simulink model "VCU_CS75_12_27_test"  (R2014a)
settings: Solver=FixedStepDiscrete  StartTime=0.0  StopTime=25  FixedStep=0.0005  RelTol=1e-3
undefined symbols (not defined in the file): D1, D2, D3, ecucoder_acal, ErrorSumMax1, ErrorSumMax2, ErrorSumMax3, I1, I2, I3, I_SW01_L, LaterlAngleCommand, LDW, P1, P2, P3, RemoteAcclPosition
libraries: simulink x913, ec5744lib x39
(part 27 of 30)

== system VCU_CS75_12_27_test/长安CS75底盘程序，20ms一次/Input/CAN1_Rx/ESP_281/ReceiveMessages/Subsystem/ESP_2 ==
  input : Inport
  Demux : Demux  Outputs=8
  ESP_ABSActiveStatus_Ad : Sum
  ESP_ABSActiveStatus_Convert : DataTypeConversion  OutDataTypeStr=uint32
  ESP_ABSActiveStatus_F : Gain
  ESP_ABSActiveStatus_L : simulink/Logic and Bit Operations/Bitwise Operator  logicop=AND  UseBitMask=on  BitMask=128  BitMaskRealWorld=Stored Integer
  ESP_ABSActiveStatus_O : Constant  Value=0  OutDataTypeStr=single
  ESP_ABSActiveStatus_S : ArithShift  BitShiftNumber=7
  ESP_ABSActiveStatus_Sub : Subsystem
  ESP_ABSActiveStatus_sat : Saturate  UpperLimit=1  LowerLimit=0
  ESP_ABSActiveStatuscv : DataTypeConversion
  ESP_ABSFailStatus_Ad : Sum
  ESP_ABSFailStatus_Convert : DataTypeConversion  OutDataTypeStr=uint32
  ESP_ABSFailStatus_F : Gain
  ESP_ABSFailStatus_L : simulink/Logic and Bit Operations/Bitwise Operator  logicop=AND  UseBitMask=on  BitMask=8  BitMaskRealWorld=Stored Integer
  ESP_ABSFailStatus_O : Constant  Value=0  OutDataTypeStr=single
  ESP_ABSFailStatus_S : ArithShift  BitShiftNumber=3
  ESP_ABSFailStatus_Sub : Subsystem
  ESP_ABSFailStatus_sat : Saturate  UpperLimit=1  LowerLimit=0
  ESP_ABSFailStatuscv : DataTypeConversion
  ESP_BrakePedalStatus_Ad : Sum
  ESP_BrakePedalStatus_Convert : DataTypeConversion  OutDataTypeStr=uint32
  ESP_BrakePedalStatus_F : Gain
  ESP_BrakePedalStatus_L : simulink/Logic and Bit Operations/Bitwise Operator  logicop=AND  UseBitMask=on  BitMask=96  BitMaskRealWorld=Stored Integer
  ESP_BrakePedalStatus_O : Constant  Value=0  OutDataTypeStr=single
  ESP_BrakePedalStatus_S : ArithShift  BitShiftNumber=5
  ESP_BrakePedalStatus_Sub : Subsystem
  ESP_BrakePedalStatus_sat : Saturate  UpperLimit=3  LowerLimit=0
  ESP_BrakePedalStatuscv : DataTypeConversion
  ESP_Checksum_Ad : Sum
  ESP_Checksum_Convert : DataTypeConversion  OutDataTypeStr=uint32
  ESP_Checksum_F : Gain
  ESP_Checksum_L : simulink/Logic and Bit Operations/Bitwise Operator  logicop=AND  UseBitMask=on  BitMask=255  BitMaskRealWorld=Stored Integer
  ESP_Checksum_O : Constant  Value=0  OutDataTypeStr=single
  ESP_Checksum_S : ArithShift
  ESP_Checksum_Sub : Subsystem
  ESP_Checksum_sat : Saturate  UpperLimit=255  LowerLimit=0
  ESP_Checksumcv : DataTypeConversion
  ESP_EBDFailStatus_Ad : Sum
  ESP_EBDFailStatus_Convert : DataTypeConversion  OutDataTypeStr=uint32
  ESP_EBDFailStatus_F : Gain
  ESP_EBDFailStatus_L : simulink/Logic and Bit Operations/Bitwise Operator  logicop=AND  UseBitMask=on  BitMask=4  BitMaskRealWorld=Stored Integer
  ESP_EBDFailStatus_O : Constant  Value=0  OutDataTypeStr=single
  ESP_EBDFailStatus_S : ArithShift  BitShiftNumber=2
  ESP_EBDFailStatus_Sub : Subsystem
  ESP_EBDFailStatus_sat : Saturate  UpperLimit=1  LowerLimit=0
  ESP_EBDFailStatuscv : DataTypeConversion
  ESP_ESPActiveStatus_Ad : Sum
  ESP_ESPActiveStatus_Convert : DataTypeConversion  OutDataTypeStr=uint32
  ESP_ESPActiveStatus_F : Gain
  ESP_ESPActiveStatus_L : simulink/Logic and Bit Operations/Bitwise Operator  logicop=AND  UseBitMask=on  BitMask=1  BitMaskRealWorld=Stored Integer
  ESP_ESPActiveStatus_O : Constant  Value=0  OutDataTypeStr=single
  ESP_ESPActiveStatus_S : ArithShift
  ESP_ESPActiveStatus_Sub : Subsystem
  ESP_ESPActiveStatus_sat : Saturate  UpperLimit=1  LowerLimit=0
  ESP_ESPActiveStatuscv : DataTypeConversion
  ESP_ESPFailStatus_Ad : Sum
  ESP_ESPFailStatus_Convert : DataTypeConversion  OutDataTypeStr=uint32
  ESP_ESPFailStatus_F : Gain
  ESP_ESPFailStatus_L : simulink/Logic and Bit Operations/Bitwise Operator  logicop=AND  UseBitMask=on  BitMask=16  BitMaskRealWorld=Stored Integer
  ESP_ESPFailStatus_O : Constant  Value=0  OutDataTypeStr=single
  ESP_ESPFailStatus_S : ArithShift  BitShiftNumber=4
  ESP_ESPFailStatus_Sub : Subsystem
  ESP_ESPFailStatus_sat : Saturate  UpperLimit=1  LowerLimit=0
  ESP_ESPFailStatuscv : DataTypeConversion
  ESP_ESPSwitchStatus_Ad : Sum
  ESP_ESPSwitchStatus_Convert : DataTypeConversion  OutDataTypeStr=uint32
  ESP_ESPSwitchStatus_F : Gain
  ESP_ESPSwitchStatus_L : simulink/Logic and Bit Operations/Bitwise Operator  logicop=AND  UseBitMask=on  BitMask=2  BitMaskRealWorld=Stored Integer
  ESP_ESPSwitchStatus_O : Constant  Value=0  OutDataTypeStr=single
  ESP_ESPSwitchStatus_S : ArithShift  BitShiftNumber=1
  ESP_ESPSwitchStatus_Sub : Subsystem
  ESP_ESPSwitchStatus_sat : Saturate  UpperLimit=1  LowerLimit=0
  ESP_ESPSwitchStatuscv : DataTypeConversion
  ESP_RollingCounter_Ad : Sum
  ESP_RollingCounter_Convert : DataTypeConversion  OutDataTypeStr=uint32
  ESP_RollingCounter_F : Gain
  ESP_RollingCounter_L : simulink/Logic and Bit Operations/Bitwise Operator  logicop=AND  UseBitMask=on  BitMask=15  BitMaskRealWorld=Stored Integer
  ESP_RollingCounter_O : Constant  Value=0  OutDataTypeStr=single
  ESP_RollingCounter_S : ArithShift
  ESP_RollingCounter_Sub : Subsystem
  ESP_RollingCounter_sat : Saturate  UpperLimit=15  LowerLimit=0
  ESP_RollingCountercv : DataTypeConversion
  ESP_VehicleSpeed_Ad : Sum
  ESP_VehicleSpeed_Convert : DataTypeConversion  OutDataTypeStr=uint32
  ESP_VehicleSpeed_F : Gain  Gain=0.05625
  ESP_VehicleSpeed_L : simulink/Logic and Bit Operations/Bitwise Operator  logicop=AND  UseBitMask=on  BitMask=8191  BitMaskRealWorld=Stored Integer
  ESP_VehicleSpeed_O : Constant  Value=0  OutDataTypeStr=single
  ESP_VehicleSpeed_S : ArithShift
  ESP_VehicleSpeed_Status_Ad : Sum
  ESP_VehicleSpeed_Status_Convert : DataTypeConversion  OutDataTypeStr=uint32
  ESP_VehicleSpeed_Status_F : Gain
  ESP_VehicleSpeed_Status_L : simulink/Logic and Bit Operations/Bitwise Operator  logicop=AND  UseBitMask=on  BitMask=32  BitMaskRealWorld=Stored Integer
  ESP_VehicleSpeed_Status_O : Constant  Value=0  OutDataTypeStr=single
  ESP_VehicleSpeed_Status_S : ArithShift  BitShiftNumber=5
  ESP_VehicleSpeed_Status_Sub : Subsystem
  ESP_VehicleSpeed_Status_sat : Saturate  UpperLimit=1  LowerLimit=0
  ESP_VehicleSpeed_Statuscv : DataTypeConversion
  ESP_VehicleSpeed_Sub : Subsystem
  ESP_VehicleSpeed_sat : Saturate  UpperLimit=360  LowerLimit=0
  ESP_VehicleSpeedcv : DataTypeConversion
  ESP_VehicleSpeedinput5_Ad : Sum
  ESP_VehicleSpeedinput5_C : Constant  Value=256
  ESP_VehicleSpeedinput5_P : Product
  ESP_ESPActiveStatus_Out : Outport
  ESP_ESPSwitchStatus_Out : Outport  Port=2
  ESP_EBDFailStatus_Out : Outport  Port=3
  ESP_ABSFailStatus_Out : Outport  Port=4
  ESP_ESPFailStatus_Out : Outport  Port=5
  ESP_ABSActiveStatus_Out : Outport  Port=6
  ESP_VehicleSpeed_Out : Outport  Port=7
  ESP_VehicleSpeed_Status_Out : Outport  Port=8
  ESP_RollingCounter_Out : Outport  Port=9
  ESP_BrakePedalStatus_Out : Outport  Port=10
  ESP_Checksum_Out : Outport  Port=11
  wires:
  input/1 -> Demux/1
  ESP_Checksumcv/1 -> ESP_Checksum_F/1
  ESP_Checksum_S/1 -> ESP_Checksumcv/1
  ESP_Checksum_L/1 -> ESP_Checksum_S/1
  ESP_Checksum_Convert/1 -> ESP_Checksum_L/1
  ESP_Checksum_Sub/1(Out1) -> ESP_Checksum_Convert/1
  Demux/8 -> ESP_Checksum_Sub/1(In1)
  ESP_Checksum_sat/1 -> ESP_Checksum_Out/1
  ESP_Checksum_Ad/1 -> ESP_Checksum_sat/1
  ESP_Checksum_O/1 -> ESP_Checksum_Ad/2
  ESP_Checksum_F/1 -> ESP_Checksum_Ad/1
  ESP_BrakePedalStatuscv/1 -> ESP_BrakePedalStatus_F/1
  ESP_BrakePedalStatus_S/1 -> ESP_BrakePedalStatuscv/1
  ESP_BrakePedalStatus_L/1 -> ESP_BrakePedalStatus_S/1
  ESP_BrakePedalStatus_Convert/1 -> ESP_BrakePedalStatus_L/1
  ESP_BrakePedalStatus_Sub/1(Out1) -> ESP_BrakePedalStatus_Convert/1
  ESP_BrakePedalStatus_sat/1 -> ESP_BrakePedalStatus_Out/1
  ESP_BrakePedalStatus_Ad/1 -> ESP_BrakePedalStatus_sat/1
  ESP_BrakePedalStatus_O/1 -> ESP_BrakePedalStatus_Ad/2
  ESP_BrakePedalStatus_F/1 -> ESP_BrakePedalStatus_Ad/1
  ESP_RollingCountercv/1 -> ESP_RollingCounter_F/1
  ESP_RollingCounter_S/1 -> ESP_RollingCountercv/1
  ESP_RollingCounter_L/1 -> ESP_RollingCounter_S/1
  ESP_RollingCounter_Convert/1 -> ESP_RollingCounter_L/1
  ESP_RollingCounter_Sub/1(Out1) -> ESP_RollingCounter_Convert/1
  Demux/7 -> ESP_BrakePedalStatus_Sub/1(In1), ESP_RollingCounter_Sub/1(In1)
  ESP_RollingCounter_sat/1 -> ESP_RollingCounter_Out/1
  ESP_RollingCounter_Ad/1 -> ESP_RollingCounter_sat/1
  ESP_RollingCounter_O/1 -> ESP_RollingCounter_Ad/2
  ESP_RollingCounter_F/1 -> ESP_RollingCounter_Ad/1
  ESP_VehicleSpeed_Statuscv/1 -> ESP_VehicleSpeed_Status_F/1
  ESP_VehicleSpeed_Status_S/1 -> ESP_VehicleSpeed_Statuscv/1
  ESP_VehicleSpeed_Status_L/1 -> ESP_VehicleSpeed_Status_S/1
  ESP_VehicleSpeed_Status_Convert/1 -> ESP_VehicleSpeed_Status_L/1
  ESP_VehicleSpeed_Status_Sub/1(Out1) -> ESP_VehicleSpeed_Status_Convert/1
  ESP_VehicleSpeed_Status_sat/1 -> ESP_VehicleSpeed_Status_Out/1
  ESP_VehicleSpeed_Status_Ad/1 -> ESP_VehicleSpeed_Status_sat/1
  ESP_VehicleSpeed_Status_O/1 -> ESP_VehicleSpeed_Status_Ad/2
  ESP_VehicleSpeed_Status_F/1 -> ESP_VehicleSpeed_Status_Ad/1
  ESP_VehicleSpeedcv/1 -> ESP_VehicleSpeed_F/1
  ESP_VehicleSpeed_S/1 -> ESP_VehicleSpeedcv/1
  ESP_VehicleSpeed_L/1 -> ESP_VehicleSpeed_S/1
  ESP_VehicleSpeed_Convert/1 -> ESP_VehicleSpeed_L/1
  ESP_VehicleSpeed_Sub/1(Out1) -> ESP_VehicleSpeed_Convert/1
  ESP_VehicleSpeedinput5_Ad/1 -> ESP_VehicleSpeed_Sub/1(In1)
  Demux/6 -> ESP_VehicleSpeedinput5_Ad/2
  ESP_VehicleSpeedinput5_P/1 -> ESP_VehicleSpeedinput5_Ad/1
  ESP_VehicleSpeedinput5_C/1 -> ESP_VehicleSpeedinput5_P/2
  Demux/5 -> ESP_VehicleSpeed_Status_Sub/1(In1), ESP_VehicleSpeedinput5_P/1
  ESP_VehicleSpeed_sat/1 -> ESP_VehicleSpeed_Out/1
  ESP_VehicleSpeed_Ad/1 -> ESP_VehicleSpeed_sat/1
  ESP_VehicleSpeed_O/1 -> ESP_VehicleSpeed_Ad/2
  ESP_VehicleSpeed_F/1 -> ESP_VehicleSpeed_Ad/1
  ESP_ABSActiveStatuscv/1 -> ESP_ABSActiveStatus_F/1
  ESP_ABSActiveStatus_S/1 -> ESP_ABSActiveStatuscv/1
  ESP_ABSActiveStatus_L/1 -> ESP_ABSActiveStatus_S/1
  ESP_ABSActiveStatus_Convert/1 -> ESP_ABSActiveStatus_L/1
  ESP_ABSActiveStatus_Sub/1(Out1) -> ESP_ABSActiveStatus_Convert/1
  ESP_ABSActiveStatus_sat/1 -> ESP_ABSActiveStatus_Out/1
  ESP_ABSActiveStatus_Ad/1 -> ESP_ABSActiveStatus_sat/1
  ESP_ABSActiveStatus_O/1 -> ESP_ABSActiveStatus_Ad/2
  ESP_ABSActiveStatus_F/1 -> ESP_ABSActiveStatus_Ad/1
  ESP_ESPFailStatuscv/1 -> ESP_ESPFailStatus_F/1
  ESP_ESPFailStatus_S/1 -> ESP_ESPFailStatuscv/1
  ESP_ESPFailStatus_L/1 -> ESP_ESPFailStatus_S/1
  ESP_ESPFailStatus_Convert/1 -> ESP_ESPFailStatus_L/1
  ESP_ESPFailStatus_Sub/1(Out1) -> ESP_ESPFailStatus_Convert/1
  ESP_ESPFailStatus_sat/1 -> ESP_ESPFailStatus_Out/1
  ESP_ESPFailStatus_Ad/1 -> ESP_ESPFailStatus_sat/1
  ESP_ESPFailStatus_O/1 -> ESP_ESPFailStatus_Ad/2
  ESP_ESPFailStatus_F/1 -> ESP_ESPFailStatus_Ad/1
  ESP_ABSFailStatuscv/1 -> ESP_ABSFailStatus_F/1
  ESP_ABSFailStatus_S/1 -> ESP_ABSFailStatuscv/1
  ESP_ABSFailStatus_L/1 -> ESP_ABSFailStatus_S/1
  ESP_ABSFailStatus_Convert/1 -> ESP_ABSFailStatus_L/1
  ESP_ABSFailStatus_Sub/1(Out1) -> ESP_ABSFailStatus_Convert/1
  ESP_ABSFailStatus_sat/1 -> ESP_ABSFailStatus_Out/1
  ESP_ABSFailStatus_Ad/1 -> ESP_ABSFailStatus_sat/1
  ESP_ABSFailStatus_O/1 -> ESP_ABSFailStatus_Ad/2
  ESP_ABSFailStatus_F/1 -> ESP_ABSFailStatus_Ad/1
  ESP_EBDFailStatuscv/1 -> ESP_EBDFailStatus_F/1
  ESP_EBDFailStatus_S/1 -> ESP_EBDFailStatuscv/1
  ESP_EBDFailStatus_L/1 -> ESP_EBDFailStatus_S/1
  ESP_EBDFailStatus_Convert/1 -> ESP_EBDFailStatus_L/1
  ESP_EBDFailStatus_Sub/1(Out1) -> ESP_EBDFailStatus_Convert/1
  ESP_EBDFailStatus_sat/1 -> ESP_EBDFailStatus_Out/1
  ESP_EBDFailStatus_Ad/1 -> ESP_EBDFailStatus_sat/1
  ESP_EBDFailStatus_O/1 -> ESP_EBDFailStatus_Ad/2
  ESP_EBDFailStatus_F/1 -> ESP_EBDFailStatus_Ad/1
  ESP_ESPSwitchStatuscv/1 -> ESP_ESPSwitchStatus_F/1
  ESP_ESPSwitchStatus_S/1 -> ESP_ESPSwitchStatuscv/1
  ESP_ESPSwitchStatus_L/1 -> ESP_ESPSwitchStatus_S/1
  ESP_ESPSwitchStatus_Convert/1 -> ESP_ESPSwitchStatus_L/1
  ESP_ESPSwitchStatus_Sub/1(Out1) -> ESP_ESPSwitchStatus_Convert/1
  ESP_ESPSwitchStatus_sat/1 -> ESP_ESPSwitchStatus_Out/1
  ESP_ESPSwitchStatus_Ad/1 -> ESP_ESPSwitchStatus_sat/1
  ESP_ESPSwitchStatus_O/1 -> ESP_ESPSwitchStatus_Ad/2
  ESP_ESPSwitchStatus_F/1 -> ESP_ESPSwitchStatus_Ad/1
  ESP_ESPActiveStatuscv/1 -> ESP_ESPActiveStatus_F/1
  ESP_ESPActiveStatus_S/1 -> ESP_ESPActiveStatuscv/1
  ESP_ESPActiveStatus_L/1 -> ESP_ESPActiveStatus_S/1
  ESP_ESPActiveStatus_Convert/1 -> ESP_ESPActiveStatus_L/1
  ESP_ESPActiveStatus_Sub/1(Out1) -> ESP_ESPActiveStatus_Convert/1
  Demux/1 -> ESP_ABSActiveStatus_Sub/1(In1), ESP_ESPFailStatus_Sub/1(In1), ESP_EBDFailStatus_Sub/1(In1), ESP_ESPSwitchStatus_Sub/1(In1), ESP_ABSFailStatus_Sub/1(In1), ESP_ESPActiveStatus_Sub/1(In1)
  ESP_ESPActiveStatus_sat/1 -> ESP_ESPActiveStatus_Out/1
  ESP_ESPActiveStatus_Ad/1 -> ESP_ESPActiveStatus_sat/1
  ESP_ESPActiveStatus_O/1 -> ESP_ESPActiveStatus_Ad/2
  ESP_ESPActiveStatus_F/1 -> ESP_ESPActiveStatus_Ad/1

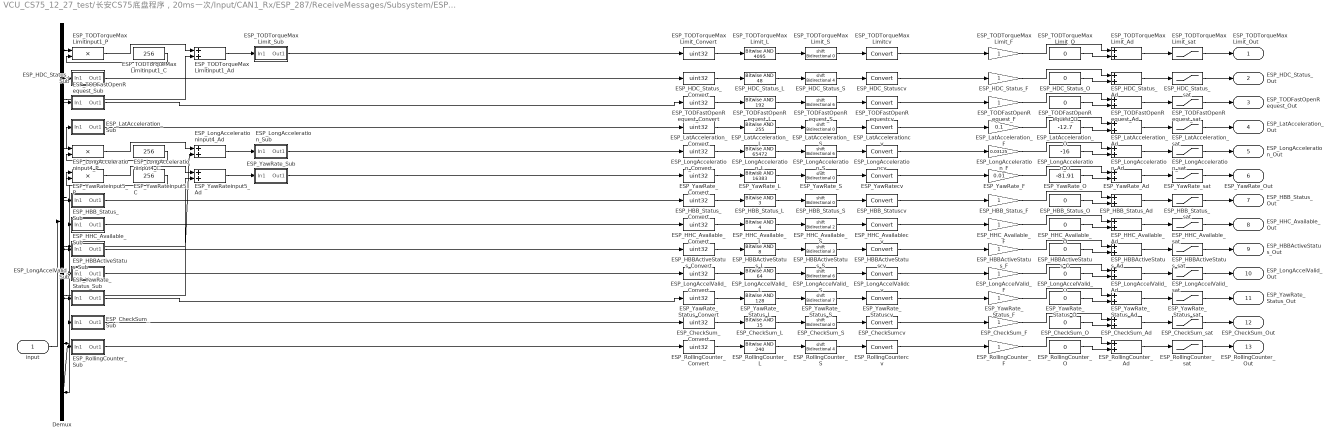
== system VCU_CS75_12_27_test/长安CS75底盘程序，20ms一次/Input/CAN1_Rx/ESP_287/ReceiveMessages/Subsystem/ESP_2 ==
  input : Inport
  Demux : Demux  Outputs=8
  ESP_CheckSum_Ad : Sum
  ESP_CheckSum_Convert : DataTypeConversion  OutDataTypeStr=uint32
  ESP_CheckSum_F : Gain
  ESP_CheckSum_L : simulink/Logic and Bit Operations/Bitwise Operator  logicop=AND  UseBitMask=on  BitMask=15  BitMaskRealWorld=Stored Integer
  ESP_CheckSum_O : Constant  Value=0  OutDataTypeStr=single
  ESP_CheckSum_S : ArithShift
  ESP_CheckSum_Sub : Subsystem
  ESP_CheckSum_sat : Saturate  UpperLimit=15  LowerLimit=0
  ESP_CheckSumcv : DataTypeConversion
  ESP_HBBActiveStatus_Ad : Sum
  ESP_HBBActiveStatus_Convert : DataTypeConversion  OutDataTypeStr=uint32
  ESP_HBBActiveStatus_F : Gain
  ESP_HBBActiveStatus_L : simulink/Logic and Bit Operations/Bitwise Operator  logicop=AND  UseBitMask=on  BitMask=8  BitMaskRealWorld=Stored Integer
  ESP_HBBActiveStatus_O : Constant  Value=0  OutDataTypeStr=single
  ESP_HBBActiveStatus_S : ArithShift  BitShiftNumber=3
  ESP_HBBActiveStatus_Sub : Subsystem
  ESP_HBBActiveStatus_sat : Saturate  UpperLimit=1  LowerLimit=0
  ESP_HBBActiveStatuscv : DataTypeConversion
  ESP_HBB_Status_Ad : Sum
  ESP_HBB_Status_Convert : DataTypeConversion  OutDataTypeStr=uint32
  ESP_HBB_Status_F : Gain
  ESP_HBB_Status_L : simulink/Logic and Bit Operations/Bitwise Operator  logicop=AND  UseBitMask=on  BitMask=3  BitMaskRealWorld=Stored Integer
  ESP_HBB_Status_O : Constant  Value=0  OutDataTypeStr=single
  ESP_HBB_Status_S : ArithShift
  ESP_HBB_Status_Sub : Subsystem
  ESP_HBB_Status_sat : Saturate  UpperLimit=3  LowerLimit=0
  ESP_HBB_Statuscv : DataTypeConversion
  ESP_HDC_Status_Ad : Sum
  ESP_HDC_Status_Convert : DataTypeConversion  OutDataTypeStr=uint32
  ESP_HDC_Status_F : Gain
  ESP_HDC_Status_L : simulink/Logic and Bit Operations/Bitwise Operator  logicop=AND  UseBitMask=on  BitMask=48  BitMaskRealWorld=Stored Integer
  ESP_HDC_Status_O : Constant  Value=0  OutDataTypeStr=single
  ESP_HDC_Status_S : ArithShift  BitShiftNumber=4
  ESP_HDC_Status_Sub : Subsystem
  ESP_HDC_Status_sat : Saturate  UpperLimit=3  LowerLimit=0
  ESP_HDC_Statuscv : DataTypeConversion
  ESP_HHC_Available_Ad : Sum
  ESP_HHC_Available_Convert : DataTypeConversion  OutDataTypeStr=uint32
  ESP_HHC_Available_F : Gain
  ESP_HHC_Available_L : simulink/Logic and Bit Operations/Bitwise Operator  logicop=AND  UseBitMask=on  BitMask=4  BitMaskRealWorld=Stored Integer
  ESP_HHC_Available_O : Constant  Value=0  OutDataTypeStr=single
  ESP_HHC_Available_S : ArithShift  BitShiftNumber=2
  ESP_HHC_Available_Sub : Subsystem
  ESP_HHC_Available_sat : Saturate  UpperLimit=1  LowerLimit=0
  ESP_HHC_Availablecv : DataTypeConversion
  ESP_LatAcceleration_Ad : Sum
  ESP_LatAcceleration_Convert : DataTypeConversion  OutDataTypeStr=uint32
  ESP_LatAcceleration_F : Gain  Gain=0.1
  ESP_LatAcceleration_L : simulink/Logic and Bit Operations/Bitwise Operator  logicop=AND  UseBitMask=on  BitMask=255  BitMaskRealWorld=Stored Integer
  ESP_LatAcceleration_O : Constant  Value=-12.7  OutDataTypeStr=single
  ESP_LatAcceleration_S : ArithShift
  ESP_LatAcceleration_Sub : Subsystem
  ESP_LatAcceleration_sat : Saturate  UpperLimit=12.7  LowerLimit=-12.7
  ESP_LatAccelerationcv : DataTypeConversion
  ESP_LongAccelValid_Ad : Sum
  ESP_LongAccelValid_Convert : DataTypeConversion  OutDataTypeStr=uint32
  ESP_LongAccelValid_F : Gain
  ESP_LongAccelValid_L : simulink/Logic and Bit Operations/Bitwise Operator  logicop=AND  UseBitMask=on  BitMask=64  BitMaskRealWorld=Stored Integer
  ESP_LongAccelValid_O : Constant  Value=0  OutDataTypeStr=single
  ESP_LongAccelValid_S : ArithShift  BitShiftNumber=6
  ESP_LongAccelValid_Sub : Subsystem
  ESP_LongAccelValid_sat : Saturate  UpperLimit=1  LowerLimit=0
  ESP_LongAccelValidcv : DataTypeConversion
  ESP_LongAcceleration_Ad : Sum
  ESP_LongAcceleration_Convert : DataTypeConversion  OutDataTypeStr=uint32
  ESP_LongAcceleration_F : Gain  Gain=0.03125
  ESP_LongAcceleration_L : simulink/Logic and Bit Operations/Bitwise Operator  logicop=AND  UseBitMask=on  BitMask=65472  BitMaskRealWorld=Stored Integer
  ESP_LongAcceleration_O : Constant  Value=-16  OutDataTypeStr=single
  ESP_LongAcceleration_S : ArithShift  BitShiftNumber=6
  ESP_LongAcceleration_Sub : Subsystem
  ESP_LongAcceleration_sat : Saturate  UpperLimit=15.96875  LowerLimit=-16
  ESP_LongAccelerationcv : DataTypeConversion
  ESP_LongAccelerationinput4_Ad : Sum
  ESP_LongAccelerationinput4_C : Constant  Value=256
  ESP_LongAccelerationinput4_P : Product
  ESP_RollingCounter_Ad : Sum
  ESP_RollingCounter_Convert : DataTypeConversion  OutDataTypeStr=uint32
  ESP_RollingCounter_F : Gain
  ESP_RollingCounter_L : simulink/Logic and Bit Operations/Bitwise Operator  logicop=AND  UseBitMask=on  BitMask=240  BitMaskRealWorld=Stored Integer
  ESP_RollingCounter_O : Constant  Value=0  OutDataTypeStr=single
  ESP_RollingCounter_S : ArithShift  BitShiftNumber=4
  ESP_RollingCounter_Sub : Subsystem
  ESP_RollingCounter_sat : Saturate  UpperLimit=15  LowerLimit=0
  ESP_RollingCountercv : DataTypeConversion
  ESP_TODFastOpenRequest_Ad : Sum
  ESP_TODFastOpenRequest_Convert : DataTypeConversion  OutDataTypeStr=uint32
  ESP_TODFastOpenRequest_F : Gain
  ESP_TODFastOpenRequest_L : simulink/Logic and Bit Operations/Bitwise Operator  logicop=AND  UseBitMask=on  BitMask=192  BitMaskRealWorld=Stored Integer
  ESP_TODFastOpenRequest_O : Constant  Value=0  OutDataTypeStr=single
  ESP_TODFastOpenRequest_S : ArithShift  BitShiftNumber=6
  ESP_TODFastOpenRequest_Sub : Subsystem
  ESP_TODFastOpenRequest_sat : Saturate  UpperLimit=3  LowerLimit=0
  ESP_TODFastOpenRequestcv : DataTypeConversion
  ESP_TODTorqueMaxLimit_Ad : Sum
  ESP_TODTorqueMaxLimit_Convert : DataTypeConversion  OutDataTypeStr=uint32
  ESP_TODTorqueMaxLimit_F : Gain
  ESP_TODTorqueMaxLimit_L : simulink/Logic and Bit Operations/Bitwise Operator  logicop=AND  UseBitMask=on  BitMask=4095  BitMaskRealWorld=Stored Integer
  ESP_TODTorqueMaxLimit_O : Constant  Value=0  OutDataTypeStr=single
  ESP_TODTorqueMaxLimit_S : ArithShift
  ESP_TODTorqueMaxLimit_Sub : Subsystem
  ESP_TODTorqueMaxLimit_sat : Saturate  UpperLimit=4095  LowerLimit=0
  ESP_TODTorqueMaxLimitcv : DataTypeConversion
  ESP_TODTorqueMaxLimitinput1_Ad : Sum
  ESP_TODTorqueMaxLimitinput1_C : Constant  Value=256
  ESP_TODTorqueMaxLimitinput1_P : Product
  ESP_YawRate_Ad : Sum
  ESP_YawRate_Convert : DataTypeConversion  OutDataTypeStr=uint32
  ESP_YawRate_F : Gain  Gain=0.01
  ESP_YawRate_L : simulink/Logic and Bit Operations/Bitwise Operator  logicop=AND  UseBitMask=on  BitMask=16383  BitMaskRealWorld=Stored Integer
  ESP_YawRate_O : Constant  Value=-81.91  OutDataTypeStr=single
  ESP_YawRate_S : ArithShift
  ESP_YawRate_Status_Ad : Sum
  ESP_YawRate_Status_Convert : DataTypeConversion  OutDataTypeStr=uint32
  ESP_YawRate_Status_F : Gain
  ESP_YawRate_Status_L : simulink/Logic and Bit Operations/Bitwise Operator  logicop=AND  UseBitMask=on  BitMask=128  BitMaskRealWorld=Stored Integer
  ESP_YawRate_Status_O : Constant  Value=0  OutDataTypeStr=single
  ESP_YawRate_Status_S : ArithShift  BitShiftNumber=7
  ESP_YawRate_Status_Sub : Subsystem
  ESP_YawRate_Status_sat : Saturate  UpperLimit=1  LowerLimit=0
  ESP_YawRate_Statuscv : DataTypeConversion
  ESP_YawRate_Sub : Subsystem
  ESP_YawRate_sat : Saturate  UpperLimit=81.91  LowerLimit=-81.91
  ESP_YawRatecv : DataTypeConversion
  ESP_YawRateinput5_Ad : Sum
  ESP_YawRateinput5_C : Constant  Value=256
  ESP_YawRateinput5_P : Product
  ESP_TODTorqueMaxLimit_Out : Outport
  ESP_HDC_Status_Out : Outport  Port=2
  ESP_TODFastOpenRequest_Out : Outport  Port=3
  ESP_LatAcceleration_Out : Outport  Port=4
  ESP_LongAcceleration_Out : Outport  Port=5
  ESP_YawRate_Out : Outport  Port=6
  ESP_HBB_Status_Out : Outport  Port=7
  ESP_HHC_Available_Out : Outport  Port=8
  ESP_HBBActiveStatus_Out : Outport  Port=9
  ESP_LongAccelValid_Out : Outport  Port=10
  ESP_YawRate_Status_Out : Outport  Port=11
  ESP_CheckSum_Out : Outport  Port=12
  ESP_RollingCounter_Out : Outport  Port=13
  wires:
  ESP_TODTorqueMaxLimit_F/1 -> ESP_TODTorqueMaxLimit_Ad/1
  ESP_TODTorqueMaxLimit_O/1 -> ESP_TODTorqueMaxLimit_Ad/2
  ESP_TODTorqueMaxLimit_Ad/1 -> ESP_TODTorqueMaxLimit_sat/1
  ESP_TODTorqueMaxLimit_sat/1 -> ESP_TODTorqueMaxLimit_Out/1
  Demux/1 -> ESP_HDC_Status_Sub/1(In1), ESP_TODFastOpenRequest_Sub/1(In1), ESP_TODTorqueMaxLimitinput1_P/1
  ESP_TODTorqueMaxLimitinput1_C/1 -> ESP_TODTorqueMaxLimitinput1_P/2
  ESP_TODTorqueMaxLimitinput1_P/1 -> ESP_TODTorqueMaxLimitinput1_Ad/1
  Demux/2 -> ESP_TODTorqueMaxLimitinput1_Ad/2
  ESP_TODTorqueMaxLimitinput1_Ad/1 -> ESP_TODTorqueMaxLimit_Sub/1(In1)
  ESP_TODTorqueMaxLimit_Sub/1(Out1) -> ESP_TODTorqueMaxLimit_Convert/1
  ESP_TODTorqueMaxLimit_Convert/1 -> ESP_TODTorqueMaxLimit_L/1
  ESP_TODTorqueMaxLimit_L/1 -> ESP_TODTorqueMaxLimit_S/1
  ESP_TODTorqueMaxLimit_S/1 -> ESP_TODTorqueMaxLimitcv/1
  ESP_TODTorqueMaxLimitcv/1 -> ESP_TODTorqueMaxLimit_F/1
  ESP_HDC_Status_F/1 -> ESP_HDC_Status_Ad/1
  ESP_HDC_Status_O/1 -> ESP_HDC_Status_Ad/2
  ESP_HDC_Status_Ad/1 -> ESP_HDC_Status_sat/1
  ESP_HDC_Status_sat/1 -> ESP_HDC_Status_Out/1
  ESP_HDC_Status_Sub/1(Out1) -> ESP_HDC_Status_Convert/1
  ESP_HDC_Status_Convert/1 -> ESP_HDC_Status_L/1
  ESP_HDC_Status_L/1 -> ESP_HDC_Status_S/1
  ESP_HDC_Status_S/1 -> ESP_HDC_Statuscv/1
  ESP_HDC_Statuscv/1 -> ESP_HDC_Status_F/1
  ESP_TODFastOpenRequest_F/1 -> ESP_TODFastOpenRequest_Ad/1
  ESP_TODFastOpenRequest_O/1 -> ESP_TODFastOpenRequest_Ad/2
  ESP_TODFastOpenRequest_Ad/1 -> ESP_TODFastOpenRequest_sat/1
  ESP_TODFastOpenRequest_sat/1 -> ESP_TODFastOpenRequest_Out/1
  ESP_TODFastOpenRequest_Sub/1(Out1) -> ESP_TODFastOpenRequest_Convert/1
  ESP_TODFastOpenRequest_Convert/1 -> ESP_TODFastOpenRequest_L/1
  ESP_TODFastOpenRequest_L/1 -> ESP_TODFastOpenRequest_S/1
  ESP_TODFastOpenRequest_S/1 -> ESP_TODFastOpenRequestcv/1
  ESP_TODFastOpenRequestcv/1 -> ESP_TODFastOpenRequest_F/1
  ESP_LatAcceleration_F/1 -> ESP_LatAcceleration_Ad/1
  ESP_LatAcceleration_O/1 -> ESP_LatAcceleration_Ad/2
  ESP_LatAcceleration_Ad/1 -> ESP_LatAcceleration_sat/1
  ESP_LatAcceleration_sat/1 -> ESP_LatAcceleration_Out/1
  Demux/3 -> ESP_LatAcceleration_Sub/1(In1)
  ESP_LatAcceleration_Sub/1(Out1) -> ESP_LatAcceleration_Convert/1
  ESP_LatAcceleration_Convert/1 -> ESP_LatAcceleration_L/1
  ESP_LatAcceleration_L/1 -> ESP_LatAcceleration_S/1
  ESP_LatAcceleration_S/1 -> ESP_LatAccelerationcv/1
  ESP_LatAccelerationcv/1 -> ESP_LatAcceleration_F/1
  ESP_LongAcceleration_F/1 -> ESP_LongAcceleration_Ad/1
  ESP_LongAcceleration_O/1 -> ESP_LongAcceleration_Ad/2
  ESP_LongAcceleration_Ad/1 -> ESP_LongAcceleration_sat/1
  ESP_LongAcceleration_sat/1 -> ESP_LongAcceleration_Out/1
  Demux/4 -> ESP_LongAccelerationinput4_P/1
  ESP_LongAccelerationinput4_C/1 -> ESP_LongAccelerationinput4_P/2
  ESP_LongAccelerationinput4_P/1 -> ESP_LongAccelerationinput4_Ad/1
  Demux/5 -> ESP_LongAccelerationinput4_Ad/2, ESP_YawRateinput5_P/1
  ESP_LongAccelerationinput4_Ad/1 -> ESP_LongAcceleration_Sub/1(In1)
  ESP_LongAcceleration_Sub/1(Out1) -> ESP_LongAcceleration_Convert/1
  ESP_LongAcceleration_Convert/1 -> ESP_LongAcceleration_L/1
  ESP_LongAcceleration_L/1 -> ESP_LongAcceleration_S/1
  ESP_LongAcceleration_S/1 -> ESP_LongAccelerationcv/1
  ESP_LongAccelerationcv/1 -> ESP_LongAcceleration_F/1
  ESP_YawRate_F/1 -> ESP_YawRate_Ad/1
  ESP_YawRate_O/1 -> ESP_YawRate_Ad/2
  ESP_YawRate_Ad/1 -> ESP_YawRate_sat/1
  ESP_YawRate_sat/1 -> ESP_YawRate_Out/1
  ESP_YawRateinput5_C/1 -> ESP_YawRateinput5_P/2
  ESP_YawRateinput5_P/1 -> ESP_YawRateinput5_Ad/1
  Demux/6 -> ESP_YawRateinput5_Ad/2
  ESP_YawRateinput5_Ad/1 -> ESP_YawRate_Sub/1(In1)
  ESP_YawRate_Sub/1(Out1) -> ESP_YawRate_Convert/1
  ESP_YawRate_Convert/1 -> ESP_YawRate_L/1
  ESP_YawRate_L/1 -> ESP_YawRate_S/1
  ESP_YawRate_S/1 -> ESP_YawRatecv/1
  ESP_YawRatecv/1 -> ESP_YawRate_F/1
  ESP_HBB_Status_F/1 -> ESP_HBB_Status_Ad/1
  ESP_HBB_Status_O/1 -> ESP_HBB_Status_Ad/2
  ESP_HBB_Status_Ad/1 -> ESP_HBB_Status_sat/1
  ESP_HBB_Status_sat/1 -> ESP_HBB_Status_Out/1
  Demux/7 -> ESP_HHC_Available_Sub/1(In1), ESP_LongAccelValid_Sub/1(In1), ESP_HBB_Status_Sub/1(In1), ESP_HBBActiveStatus_Sub/1(In1), ESP_YawRate_Status_Sub/1(In1)
  ESP_HBB_Status_Sub/1(Out1) -> ESP_HBB_Status_Convert/1
  ESP_HBB_Status_Convert/1 -> ESP_HBB_Status_L/1
  ESP_HBB_Status_L/1 -> ESP_HBB_Status_S/1
  ESP_HBB_Status_S/1 -> ESP_HBB_Statuscv/1
  ESP_HBB_Statuscv/1 -> ESP_HBB_Status_F/1
  ESP_HHC_Available_F/1 -> ESP_HHC_Available_Ad/1
  ESP_HHC_Available_O/1 -> ESP_HHC_Available_Ad/2
  ESP_HHC_Available_Ad/1 -> ESP_HHC_Available_sat/1
  ESP_HHC_Available_sat/1 -> ESP_HHC_Available_Out/1
  ESP_HHC_Available_Sub/1(Out1) -> ESP_HHC_Available_Convert/1
  ESP_HHC_Available_Convert/1 -> ESP_HHC_Available_L/1
  ESP_HHC_Available_L/1 -> ESP_HHC_Available_S/1
  ESP_HHC_Available_S/1 -> ESP_HHC_Availablecv/1
  ESP_HHC_Availablecv/1 -> ESP_HHC_Available_F/1
  ESP_HBBActiveStatus_F/1 -> ESP_HBBActiveStatus_Ad/1
  ESP_HBBActiveStatus_O/1 -> ESP_HBBActiveStatus_Ad/2
  ESP_HBBActiveStatus_Ad/1 -> ESP_HBBActiveStatus_sat/1
  ESP_HBBActiveStatus_sat/1 -> ESP_HBBActiveStatus_Out/1
  ESP_HBBActiveStatus_Sub/1(Out1) -> ESP_HBBActiveStatus_Convert/1
  ESP_HBBActiveStatus_Convert/1 -> ESP_HBBActiveStatus_L/1
  ESP_HBBActiveStatus_L/1 -> ESP_HBBActiveStatus_S/1
  ESP_HBBActiveStatus_S/1 -> ESP_HBBActiveStatuscv/1
  ESP_HBBActiveStatuscv/1 -> ESP_HBBActiveStatus_F/1
  ESP_LongAccelValid_F/1 -> ESP_LongAccelValid_Ad/1
  ESP_LongAccelValid_O/1 -> ESP_LongAccelValid_Ad/2
  ESP_LongAccelValid_Ad/1 -> ESP_LongAccelValid_sat/1
  ESP_LongAccelValid_sat/1 -> ESP_LongAccelValid_Out/1
  ESP_LongAccelValid_Sub/1(Out1) -> ESP_LongAccelValid_Convert/1
  ESP_LongAccelValid_Convert/1 -> ESP_LongAccelValid_L/1
  ESP_LongAccelValid_L/1 -> ESP_LongAccelValid_S/1
  ESP_LongAccelValid_S/1 -> ESP_LongAccelValidcv/1
  ESP_LongAccelValidcv/1 -> ESP_LongAccelValid_F/1
  ESP_YawRate_Status_F/1 -> ESP_YawRate_Status_Ad/1
  ESP_YawRate_Status_O/1 -> ESP_YawRate_Status_Ad/2
  ESP_YawRate_Status_Ad/1 -> ESP_YawRate_Status_sat/1
  ESP_YawRate_Status_sat/1 -> ESP_YawRate_Status_Out/1
  ESP_YawRate_Status_Sub/1(Out1) -> ESP_YawRate_Status_Convert/1
  ESP_YawRate_Status_Convert/1 -> ESP_YawRate_Status_L/1
  ESP_YawRate_Status_L/1 -> ESP_YawRate_Status_S/1
  ESP_YawRate_Status_S/1 -> ESP_YawRate_Statuscv/1
  ESP_YawRate_Statuscv/1 -> ESP_YawRate_Status_F/1
  ESP_CheckSum_F/1 -> ESP_CheckSum_Ad/1
  ESP_CheckSum_O/1 -> ESP_CheckSum_Ad/2
  ESP_CheckSum_Ad/1 -> ESP_CheckSum_sat/1
  ESP_CheckSum_sat/1 -> ESP_CheckSum_Out/1
  Demux/8 -> ESP_CheckSum_Sub/1(In1), ESP_RollingCounter_Sub/1(In1)
  ESP_CheckSum_Sub/1(Out1) -> ESP_CheckSum_Convert/1
  ESP_CheckSum_Convert/1 -> ESP_CheckSum_L/1
  ESP_CheckSum_L/1 -> ESP_CheckSum_S/1
  ESP_CheckSum_S/1 -> ESP_CheckSumcv/1
  ESP_CheckSumcv/1 -> ESP_CheckSum_F/1
  ESP_RollingCounter_F/1 -> ESP_RollingCounter_Ad/1
  ESP_RollingCounter_O/1 -> ESP_RollingCounter_Ad/2
  ESP_RollingCounter_Ad/1 -> ESP_RollingCounter_sat/1
  ESP_RollingCounter_sat/1 -> ESP_RollingCounter_Out/1
  ESP_RollingCounter_Sub/1(Out1) -> ESP_RollingCounter_Convert/1
  ESP_RollingCounter_Convert/1 -> ESP_RollingCounter_L/1
  ESP_RollingCounter_L/1 -> ESP_RollingCounter_S/1
  ESP_RollingCounter_S/1 -> ESP_RollingCountercv/1
  ESP_RollingCountercv/1 -> ESP_RollingCounter_F/1
  input/1 -> Demux/1

== system VCU_CS75_12_27_test/长安CS75底盘程序，20ms一次/Input/CAN1_Rx/GW_20B/ReceiveMessages/Subsystem/GW_20B2 ==
  input : Inport
  Data Type Conversion : DataTypeConversion
  Demux : Demux  Outputs=8
  EMS_BrakePedalStatus_Ad : Sum
  EMS_BrakePedalStatus_Convert : DataTypeConversion  OutDataTypeStr=uint32
  EMS_BrakePedalStatus_F : Gain
  EMS_BrakePedalStatus_L : simulink/Logic and Bit Operations/Bitwise Operator  logicop=AND  UseBitMask=on  BitMask=192  BitMaskRealWorld=Stored Integer
  EMS_BrakePedalStatus_O : Constant  Value=0  OutDataTypeStr=single
  EMS_BrakePedalStatus_S : ArithShift  BitShiftNumber=6
  EMS_BrakePedalStatus_Sub : Subsystem
  EMS_BrakePedalStatus_sat : Saturate  UpperLimit=3  LowerLimit=0
  EMS_BrakePedalStatuscv : DataTypeConversion
  EMS_EngineStartupEnd_Ad : Sum
  EMS_EngineStartupEnd_Convert : DataTypeConversion  OutDataTypeStr=uint32
  EMS_EngineStartupEnd_F : Gain
  EMS_EngineStartupEnd_L : simulink/Logic and Bit Operations/Bitwise Operator  logicop=AND  UseBitMask=on  BitMask=48  BitMaskRealWorld=Stored Integer
  EMS_EngineStartupEnd_O : Constant  Value=0  OutDataTypeStr=single
  EMS_EngineStartupEnd_S : ArithShift  BitShiftNumber=4
  EMS_EngineStartupEnd_Sub : Subsystem
  EMS_EngineStartupEnd_sat : Saturate  UpperLimit=3  LowerLimit=0
  EMS_EngineStartupEndcv : DataTypeConversion
  EMS_EngineStatus_Ad : Sum
  EMS_EngineStatus_Convert : DataTypeConversion  OutDataTypeStr=uint32
  EMS_EngineStatus_F : Gain
  EMS_EngineStatus_L : simulink/Logic and Bit Operations/Bitwise Operator  logicop=AND  UseBitMask=on  BitMask=48  BitMaskRealWorld=Stored Integer
  EMS_EngineStatus_O : Constant  Value=0  OutDataTypeStr=single
  EMS_EngineStatus_S : ArithShift  BitShiftNumber=4
  EMS_EngineStatus_Sub : Subsystem
  EMS_EngineStatus_sat : Saturate  UpperLimit=3  LowerLimit=0
  EMS_EngineStatuscv : DataTypeConversion
  EPB_BrakeLightOnRequest_Ad : Sum
  EPB_BrakeLightOnRequest_Convert : DataTypeConversion  OutDataTypeStr=uint32
  EPB_BrakeLightOnRequest_F : Gain
  EPB_BrakeLightOnRequest_L : simulink/Logic and Bit Operations/Bitwise Operator  logicop=AND  UseBitMask=on  BitMask=6  BitMaskRealWorld=Stored Integer
  EPB_BrakeLightOnRequest_O : Constant  Value=0  OutDataTypeStr=single
  EPB_BrakeLightOnRequest_S : ArithShift  BitShiftNumber=1
  EPB_BrakeLightOnRequest_Sub : Subsystem
  EPB_BrakeLightOnRequest_sat : Saturate  UpperLimit=3  LowerLimit=0
  EPB_BrakeLightOnRequestcv : DataTypeConversion
  EPB_Status_Ad : Sum
  EPB_Status_Convert : DataTypeConversion  OutDataTypeStr=uint32
  EPB_Status_F : Gain
  EPB_Status_L : simulink/Logic and Bit Operations/Bitwise Operator  logicop=AND  UseBitMask=on  BitMask=192  BitMaskRealWorld=Stored Integer
  EPB_Status_O : Constant  Value=0  OutDataTypeStr=single
  EPB_Status_S : ArithShift  BitShiftNumber=6
  EPB_Status_Sub : Subsystem
  EPB_Status_sat : Saturate  UpperLimit=3  LowerLimit=0
  EPB_Statuscv : DataTypeConversion
  SAS_SteeringAngleCS : ArithShift  BitShiftNumber=-16
  SAS_SteeringAngleCS1 : ArithShift  BitShiftNumber=-15
  SAS_SteeringAngleConS : Constant  OutDataTypeStr=single
  SAS_SteeringAngleMinus : UnaryMinus
  SAS_SteeringAngleROP : RelationalOperator  OutDataTypeStr=boolean
  SAS_SteeringAngleSW : Switch  Criteria=u2 ~= 0
  SAS_SteeringAngleValid_Ad : Sum
  SAS_SteeringAngleValid_Convert : DataTypeConversion  OutDataTypeStr=uint32
  SAS_SteeringAngleValid_F : Gain
  SAS_SteeringAngleValid_L : simulink/Logic and Bit Operations/Bitwise Operator  logicop=AND  UseBitMask=on  BitMask=1  BitMaskRealWorld=Stored Integer
  SAS_SteeringAngleValid_O : Constant  Value=0  OutDataTypeStr=single
  SAS_SteeringAngleValid_S : ArithShift
  SAS_SteeringAngleValid_Sub : Subsystem
  SAS_SteeringAngleValid_sat : Saturate  UpperLimit=1  LowerLimit=0
  SAS_SteeringAngleValidcv : DataTypeConversion
  SAS_SteeringAngle_Ad : Sum
  SAS_SteeringAngle_Convert : DataTypeConversion  OutDataTypeStr=uint32
  SAS_SteeringAngle_F : Gain  Gain=0.1
  SAS_SteeringAngle_L : simulink/Logic and Bit Operations/Bitwise Operator  logicop=AND  UseBitMask=on  BitMask=65535  BitMaskRealWorld=Stored Integer
  SAS_SteeringAngle_O : Constant  Value=0  OutDataTypeStr=single
  SAS_SteeringAngle_S : ArithShift
  SAS_SteeringAngle_Sub : Subsystem
  SAS_SteeringAngle_sat : Saturate  UpperLimit=780  LowerLimit=-780
  SAS_SteeringAnglecv : DataTypeConversion
  SAS_SteeringAngleinput4_Ad : Sum
  SAS_SteeringAngleinput4_C : Constant  Value=256
  SAS_SteeringAngleinput4_P : Product
  SAS_SteeringAnglesubcon : Sum  Inputs=+-
  TCU_GearShiftPositon_Ad : Sum
  TCU_GearShiftPositon_Convert : DataTypeConversion  OutDataTypeStr=uint32
  TCU_GearShiftPositon_F : Gain
  TCU_GearShiftPositon_L : simulink/Logic and Bit Operations/Bitwise Operator  logicop=AND  UseBitMask=on  BitMask=120  BitMaskRealWorld=Stored Integer
  TCU_GearShiftPositon_O : Constant  Value=0  OutDataTypeStr=single
  TCU_GearShiftPositon_S : ArithShift  BitShiftNumber=3
  TCU_GearShiftPositon_Sub : Subsystem
  TCU_GearShiftPositon_sat : Saturate  UpperLimit=15  LowerLimit=0
  TCU_GearShiftPositoncv : DataTypeConversion
  TCU_ShiftPostionValid_Ad : Sum
  TCU_ShiftPostionValid_Convert : DataTypeConversion  OutDataTypeStr=uint32
  TCU_ShiftPostionValid_F : Gain
  TCU_ShiftPostionValid_L : simulink/Logic and Bit Operations/Bitwise Operator  logicop=AND  UseBitMask=on  BitMask=128  BitMaskRealWorld=Stored Integer
  TCU_ShiftPostionValid_O : Constant  Value=0  OutDataTypeStr=single
  TCU_ShiftPostionValid_S : ArithShift  BitShiftNumber=7
  TCU_ShiftPostionValid_Sub : Subsystem
  TCU_ShiftPostionValid_sat : Saturate  UpperLimit=1  LowerLimit=0
  TCU_ShiftPostionValidcv : DataTypeConversion
  SAS_SteeringAngleValid_Out : Outport
  EMS_EngineStatus_Out : Outport  Port=2
  EMS_BrakePedalStatus_Out : Outport  Port=3
  EMS_EngineStartupEnd_Out : Outport  Port=4
  SAS_SteeringAngle_Out : Outport  Port=5
  EPB_BrakeLightOnRequest_Out : Outport  Port=6
  TCU_GearShiftPositon_Out : Outport  Port=7
  TCU_ShiftPostionValid_Out : Outport  Port=8
  EPB_Status_Out : Outport  Port=9
  wires:
  SAS_SteeringAngleValid_F/1 -> SAS_SteeringAngleValid_Ad/1
  SAS_SteeringAngleValid_O/1 -> SAS_SteeringAngleValid_Ad/2
  SAS_SteeringAngleValid_Ad/1 -> SAS_SteeringAngleValid_sat/1
  SAS_SteeringAngleValid_sat/1 -> SAS_SteeringAngleValid_Out/1
  Demux/1 -> SAS_SteeringAngleValid_Sub/1(In1), EMS_EngineStatus_Sub/1(In1), EMS_BrakePedalStatus_Sub/1(In1)
  SAS_SteeringAngleValid_Sub/1(Out1) -> SAS_SteeringAngleValid_Convert/1
  SAS_SteeringAngleValid_Convert/1 -> SAS_SteeringAngleValid_L/1
  SAS_SteeringAngleValid_L/1 -> SAS_SteeringAngleValid_S/1
  SAS_SteeringAngleValid_S/1 -> SAS_SteeringAngleValidcv/1
  SAS_SteeringAngleValidcv/1 -> SAS_SteeringAngleValid_F/1
  EMS_EngineStatus_F/1 -> EMS_EngineStatus_Ad/1
  EMS_EngineStatus_O/1 -> EMS_EngineStatus_Ad/2
  EMS_EngineStatus_Ad/1 -> EMS_EngineStatus_sat/1
  EMS_EngineStatus_sat/1 -> EMS_EngineStatus_Out/1
  EMS_EngineStatus_Sub/1(Out1) -> EMS_EngineStatus_Convert/1
  EMS_EngineStatus_Convert/1 -> EMS_EngineStatus_L/1
  EMS_EngineStatus_L/1 -> EMS_EngineStatus_S/1
  EMS_EngineStatus_S/1 -> EMS_EngineStatuscv/1
  EMS_EngineStatuscv/1 -> EMS_EngineStatus_F/1
  EMS_BrakePedalStatus_F/1 -> EMS_BrakePedalStatus_Ad/1
  EMS_BrakePedalStatus_O/1 -> EMS_BrakePedalStatus_Ad/2
  EMS_BrakePedalStatus_Ad/1 -> EMS_BrakePedalStatus_sat/1
  EMS_BrakePedalStatus_sat/1 -> EMS_BrakePedalStatus_Out/1
  EMS_BrakePedalStatus_Sub/1(Out1) -> EMS_BrakePedalStatus_Convert/1
  EMS_BrakePedalStatus_Convert/1 -> EMS_BrakePedalStatus_L/1
  EMS_BrakePedalStatus_L/1 -> EMS_BrakePedalStatus_S/1
  EMS_BrakePedalStatus_S/1 -> EMS_BrakePedalStatuscv/1
  EMS_BrakePedalStatuscv/1 -> EMS_BrakePedalStatus_F/1
  EMS_EngineStartupEnd_F/1 -> EMS_EngineStartupEnd_Ad/1
  EMS_EngineStartupEnd_O/1 -> EMS_EngineStartupEnd_Ad/2
  EMS_EngineStartupEnd_Ad/1 -> EMS_EngineStartupEnd_sat/1
  EMS_EngineStartupEnd_sat/1 -> EMS_EngineStartupEnd_Out/1
  Demux/2 -> EMS_EngineStartupEnd_Sub/1(In1)
  EMS_EngineStartupEnd_Sub/1(Out1) -> EMS_EngineStartupEnd_Convert/1
  EMS_EngineStartupEnd_Convert/1 -> EMS_EngineStartupEnd_L/1
  EMS_EngineStartupEnd_L/1 -> EMS_EngineStartupEnd_S/1
  EMS_EngineStartupEnd_S/1 -> EMS_EngineStartupEndcv/1
  EMS_EngineStartupEndcv/1 -> EMS_EngineStartupEnd_F/1
  SAS_SteeringAngle_F/1 -> SAS_SteeringAngle_Ad/1
  SAS_SteeringAngle_O/1 -> SAS_SteeringAngle_Ad/2
  SAS_SteeringAngle_Ad/1 -> SAS_SteeringAngle_sat/1
  SAS_SteeringAngle_sat/1 -> SAS_SteeringAngle_Out/1
  Demux/4 -> SAS_SteeringAngleinput4_P/1
  SAS_SteeringAngleinput4_C/1 -> SAS_SteeringAngleinput4_P/2
  SAS_SteeringAngleinput4_P/1 -> SAS_SteeringAngleinput4_Ad/1
  Demux/5 -> SAS_SteeringAngleinput4_Ad/2
  SAS_SteeringAngleinput4_Ad/1 -> SAS_SteeringAngle_Sub/1(In1)
  SAS_SteeringAngle_Sub/1(Out1) -> SAS_SteeringAngle_Convert/1
  SAS_SteeringAngle_Convert/1 -> SAS_SteeringAngle_L/1
  SAS_SteeringAngle_L/1 -> SAS_SteeringAngle_S/1
  SAS_SteeringAngle_S/1 -> SAS_SteeringAnglecv/1
  SAS_SteeringAnglecv/1 -> SAS_SteeringAngleROP/1, SAS_SteeringAnglesubcon/2, SAS_SteeringAngleSW/3
  SAS_SteeringAngleConS/1 -> SAS_SteeringAngleCS/1, SAS_SteeringAngleCS1/1
  SAS_SteeringAngleCS1/1 -> SAS_SteeringAngleROP/2
  SAS_SteeringAngleCS/1 -> SAS_SteeringAnglesubcon/1
  SAS_SteeringAnglesubcon/1 -> SAS_SteeringAngleMinus/1
  SAS_SteeringAngleMinus/1 -> SAS_SteeringAngleSW/1
  SAS_SteeringAngleSW/1 -> Data Type Conversion/1
  SAS_SteeringAngleROP/1 -> SAS_SteeringAngleSW/2
  EPB_BrakeLightOnRequest_F/1 -> EPB_BrakeLightOnRequest_Ad/1
  EPB_BrakeLightOnRequest_O/1 -> EPB_BrakeLightOnRequest_Ad/2
  EPB_BrakeLightOnRequest_Ad/1 -> EPB_BrakeLightOnRequest_sat/1
  EPB_BrakeLightOnRequest_sat/1 -> EPB_BrakeLightOnRequest_Out/1
  Demux/6 -> EPB_BrakeLightOnRequest_Sub/1(In1), TCU_GearShiftPositon_Sub/1(In1), TCU_ShiftPostionValid_Sub/1(In1)
  EPB_BrakeLightOnRequest_Sub/1(Out1) -> EPB_BrakeLightOnRequest_Convert/1
  EPB_BrakeLightOnRequest_Convert/1 -> EPB_BrakeLightOnRequest_L/1
  EPB_BrakeLightOnRequest_L/1 -> EPB_BrakeLightOnRequest_S/1
  EPB_BrakeLightOnRequest_S/1 -> EPB_BrakeLightOnRequestcv/1
  EPB_BrakeLightOnRequestcv/1 -> EPB_BrakeLightOnRequest_F/1
  TCU_GearShiftPositon_F/1 -> TCU_GearShiftPositon_Ad/1
  TCU_GearShiftPositon_O/1 -> TCU_GearShiftPositon_Ad/2
  TCU_GearShiftPositon_Ad/1 -> TCU_GearShiftPositon_sat/1
  TCU_GearShiftPositon_sat/1 -> TCU_GearShiftPositon_Out/1
  TCU_GearShiftPositon_Sub/1(Out1) -> TCU_GearShiftPositon_Convert/1
  TCU_GearShiftPositon_Convert/1 -> TCU_GearShiftPositon_L/1
  TCU_GearShiftPositon_L/1 -> TCU_GearShiftPositon_S/1
  TCU_GearShiftPositon_S/1 -> TCU_GearShiftPositoncv/1
  TCU_GearShiftPositoncv/1 -> TCU_GearShiftPositon_F/1
  TCU_ShiftPostionValid_F/1 -> TCU_ShiftPostionValid_Ad/1
  TCU_ShiftPostionValid_O/1 -> TCU_ShiftPostionValid_Ad/2
  TCU_ShiftPostionValid_Ad/1 -> TCU_ShiftPostionValid_sat/1
  TCU_ShiftPostionValid_sat/1 -> TCU_ShiftPostionValid_Out/1
  TCU_ShiftPostionValid_Sub/1(Out1) -> TCU_ShiftPostionValid_Convert/1
  TCU_ShiftPostionValid_Convert/1 -> TCU_ShiftPostionValid_L/1
  TCU_ShiftPostionValid_L/1 -> TCU_ShiftPostionValid_S/1
  TCU_ShiftPostionValid_S/1 -> TCU_ShiftPostionValidcv/1
  TCU_ShiftPostionValidcv/1 -> TCU_ShiftPostionValid_F/1
  EPB_Status_F/1 -> EPB_Status_Ad/1
  EPB_Status_O/1 -> EPB_Status_Ad/2
  EPB_Status_Ad/1 -> EPB_Status_sat/1
  EPB_Status_sat/1 -> EPB_Status_Out/1
  Demux/7 -> EPB_Status_Sub/1(In1)
  EPB_Status_Sub/1(Out1) -> EPB_Status_Convert/1
  EPB_Status_Convert/1 -> EPB_Status_L/1
  EPB_Status_L/1 -> EPB_Status_S/1
  EPB_Status_S/1 -> EPB_Statuscv/1
  EPB_Statuscv/1 -> EPB_Status_F/1
  input/1 -> Demux/1
  Data Type Conversion/1 -> SAS_SteeringAngle_F/1

== system VCU_CS75_12_27_test/长安CS75底盘程序，20ms一次/Input/CAN1_Rx/GW_308/ReceiveMessages/Subsystem/GW_1 ==
  input : Inport
  Demux : Demux  Outputs=8
  IP_TotalOdometer_Ad : Sum
  IP_TotalOdometer_Convert : DataTypeConversion  OutDataTypeStr=uint32
  IP_TotalOdometer_F : Gain  Gain=0.1
  IP_TotalOdometer_L : simulink/Logic and Bit Operations/Bitwise Operator  logicop=AND  UseBitMask=on  BitMask=16777215  BitMaskRealWorld=Stored Integer
  IP_TotalOdometer_O : Constant  Value=0  OutDataTypeStr=single
  IP_TotalOdometer_S : ArithShift
  IP_TotalOdometer_Sub : Subsystem
  IP_TotalOdometer_sat : Saturate  UpperLimit=999999  LowerLimit=0
  IP_TotalOdometercv : DataTypeConversion
  IP_TotalOdometerinput5_Ad : Sum
  IP_TotalOdometerinput5_C : Constant  Value=65536
  IP_TotalOdometerinput5_P : Product
  IP_TotalOdometerinput6_Ad : Sum
  IP_TotalOdometerinput6_C : Constant  Value=256
  IP_TotalOdometerinput6_P : Product
  IP_TotalOdometer_Out : Outport
  wires:
  input/1 -> Demux/1
  IP_TotalOdometercv/1 -> IP_TotalOdometer_F/1
  IP_TotalOdometer_S/1 -> IP_TotalOdometercv/1
  IP_TotalOdometer_L/1 -> IP_TotalOdometer_S/1
  IP_TotalOdometer_Convert/1 -> IP_TotalOdometer_L/1
  IP_TotalOdometer_Sub/1(Out1) -> IP_TotalOdometer_Convert/1
  IP_TotalOdometerinput6_Ad/1 -> IP_TotalOdometer_Sub/1(In1)
  IP_TotalOdometerinput5_Ad/1 -> IP_TotalOdometerinput6_Ad/2
  IP_TotalOdometerinput6_P/1 -> IP_TotalOdometerinput6_Ad/1
  IP_TotalOdometerinput6_C/1 -> IP_TotalOdometerinput6_P/2
  Demux/6 -> IP_TotalOdometerinput6_P/1
  Demux/7 -> IP_TotalOdometerinput5_Ad/2
  IP_TotalOdometerinput5_P/1 -> IP_TotalOdometerinput5_Ad/1
  IP_TotalOdometerinput5_C/1 -> IP_TotalOdometerinput5_P/2
  Demux/5 -> IP_TotalOdometerinput5_P/1
  IP_TotalOdometer_sat/1 -> IP_TotalOdometer_Out/1
  IP_TotalOdometer_Ad/1 -> IP_TotalOdometer_sat/1
  IP_TotalOdometer_O/1 -> IP_TotalOdometer_Ad/2
  IP_TotalOdometer_F/1 -> IP_TotalOdometer_Ad/1

== system VCU_CS75_12_27_test/长安CS75底盘程序，20ms一次/Input/CAN1_Rx/GW_332/ReceiveMessages/Subsystem/GW_1 ==
  input : Inport
  Demux : Demux  Outputs=8
  EMS_EngineSpeed_Ad : Sum
  EMS_EngineSpeed_Convert : DataTypeConversion  OutDataTypeStr=uint32
  EMS_EngineSpeed_F : Gain  Gain=0.25
  EMS_EngineSpeed_L : simulink/Logic and Bit Operations/Bitwise Operator  logicop=AND  UseBitMask=on  BitMask=65535  BitMaskRealWorld=Stored Integer
  EMS_EngineSpeed_O : Constant  Value=0  OutDataTypeStr=single
  EMS_EngineSpeed_S : ArithShift
  EMS_EngineSpeed_Sub : Subsystem
  EMS_EngineSpeed_sat : Saturate  UpperLimit=16383.5  LowerLimit=0
  EMS_EngineSpeedcv : DataTypeConversion
  EMS_EngineSpeedinput6_Ad : Sum
  EMS_EngineSpeedinput6_C : Constant  Value=256
  EMS_EngineSpeedinput6_P : Product
  SAS_SASFailure_Ad : Sum
  SAS_SASFailure_Convert : DataTypeConversion  OutDataTypeStr=uint32
  SAS_SASFailure_F : Gain
  SAS_SASFailure_L : simulink/Logic and Bit Operations/Bitwise Operator  logicop=AND  UseBitMask=on  BitMask=16  BitMaskRealWorld=Stored Integer
  SAS_SASFailure_O : Constant  Value=0  OutDataTypeStr=single
  SAS_SASFailure_S : ArithShift  BitShiftNumber=4
  SAS_SASFailure_Sub : Subsystem
  SAS_SASFailure_sat : Saturate  UpperLimit=1  LowerLimit=0
  SAS_SASFailurecv : DataTypeConversion
  SRS_DriverBuckleSwitchStatus_Ad : Sum
  SRS_DriverBuckleSwitchStatus_Convert : DataTypeConversion  OutDataTypeStr=uint32
  SRS_DriverBuckleSwitchStatus_F : Gain
  SRS_DriverBuckleSwitchStatus_L : simulink/Logic and Bit Operations/Bitwise Operator  logicop=AND  UseBitMask=on  BitMask=192  BitMaskRealWorld=Stored Integer
  SRS_DriverBuckleSwitchStatus_O : Constant  Value=0  OutDataTypeStr=single
  SRS_DriverBuckleSwitchStatus_S : ArithShift  BitShiftNumber=6
  SRS_DriverBuckleSwitchStatus_Sub : Subsystem
  SRS_DriverBuckleSwitchStatus_sat : Saturate  UpperLimit=3  LowerLimit=0
  SRS_DriverBuckleSwitchStatuscv : DataTypeConversion
  SRS_PassengerBuckleSwitchStatus_Ad : Sum
  SRS_PassengerBuckleSwitchStatus_Convert : DataTypeConversion  OutDataTypeStr=uint32
  SRS_PassengerBuckleSwitchStatus_F : Gain
  SRS_PassengerBuckleSwitchStatus_L : simulink/Logic and Bit Operations/Bitwise Operator  logicop=AND  UseBitMask=on  BitMask=48  BitMaskRealWorld=Stored Integer
  SRS_PassengerBuckleSwitchStatus_O : Constant  Value=0  OutDataTypeStr=single
  SRS_PassengerBuckleSwitchStatus_S : ArithShift  BitShiftNumber=4
  SRS_PassengerBuckleSwitchStatus_Sub : Subsystem
  SRS_PassengerBuckleSwitchStatus_sat : Saturate  UpperLimit=3  LowerLimit=0
  SRS_PassengerBuckleSwitchStatuscv : DataTypeConversion
  SRS_PassengerBuckleSwitchStatus_Out : Outport
  SRS_DriverBuckleSwitchStatus_Out : Outport  Port=2
  SAS_SASFailure_Out : Outport  Port=3
  EMS_EngineSpeed_Out : Outport  Port=4
  wires:
  input/1 -> Demux/1
  EMS_EngineSpeedcv/1 -> EMS_EngineSpeed_F/1
  EMS_EngineSpeed_S/1 -> EMS_EngineSpeedcv/1
  EMS_EngineSpeed_L/1 -> EMS_EngineSpeed_S/1
  EMS_EngineSpeed_Convert/1 -> EMS_EngineSpeed_L/1
  EMS_EngineSpeed_Sub/1(Out1) -> EMS_EngineSpeed_Convert/1
  EMS_EngineSpeedinput6_Ad/1 -> EMS_EngineSpeed_Sub/1(In1)
  Demux/7 -> EMS_EngineSpeedinput6_Ad/2
  EMS_EngineSpeedinput6_P/1 -> EMS_EngineSpeedinput6_Ad/1
  EMS_EngineSpeedinput6_C/1 -> EMS_EngineSpeedinput6_P/2
  Demux/6 -> EMS_EngineSpeedinput6_P/1
  EMS_EngineSpeed_sat/1 -> EMS_EngineSpeed_Out/1
  EMS_EngineSpeed_Ad/1 -> EMS_EngineSpeed_sat/1
  EMS_EngineSpeed_O/1 -> EMS_EngineSpeed_Ad/2
  EMS_EngineSpeed_F/1 -> EMS_EngineSpeed_Ad/1
  SAS_SASFailurecv/1 -> SAS_SASFailure_F/1
  SAS_SASFailure_S/1 -> SAS_SASFailurecv/1
  SAS_SASFailure_L/1 -> SAS_SASFailure_S/1
  SAS_SASFailure_Convert/1 -> SAS_SASFailure_L/1
  SAS_SASFailure_Sub/1(Out1) -> SAS_SASFailure_Convert/1
  Demux/5 -> SAS_SASFailure_Sub/1(In1)
  SAS_SASFailure_sat/1 -> SAS_SASFailure_Out/1
  SAS_SASFailure_Ad/1 -> SAS_SASFailure_sat/1
  SAS_SASFailure_O/1 -> SAS_SASFailure_Ad/2
  SAS_SASFailure_F/1 -> SAS_SASFailure_Ad/1
  SRS_DriverBuckleSwitchStatuscv/1 -> SRS_DriverBuckleSwitchStatus_F/1
  SRS_DriverBuckleSwitchStatus_S/1 -> SRS_DriverBuckleSwitchStatuscv/1
  SRS_DriverBuckleSwitchStatus_L/1 -> SRS_DriverBuckleSwitchStatus_S/1
  SRS_DriverBuckleSwitchStatus_Convert/1 -> SRS_DriverBuckleSwitchStatus_L/1
  SRS_DriverBuckleSwitchStatus_Sub/1(Out1) -> SRS_DriverBuckleSwitchStatus_Convert/1
  SRS_DriverBuckleSwitchStatus_sat/1 -> SRS_DriverBuckleSwitchStatus_Out/1
  SRS_DriverBuckleSwitchStatus_Ad/1 -> SRS_DriverBuckleSwitchStatus_sat/1
  SRS_DriverBuckleSwitchStatus_O/1 -> SRS_DriverBuckleSwitchStatus_Ad/2
  SRS_DriverBuckleSwitchStatus_F/1 -> SRS_DriverBuckleSwitchStatus_Ad/1
  SRS_PassengerBuckleSwitchStatuscv/1 -> SRS_PassengerBuckleSwitchStatus_F/1
  SRS_PassengerBuckleSwitchStatus_S/1 -> SRS_PassengerBuckleSwitchStatuscv/1
  SRS_PassengerBuckleSwitchStatus_L/1 -> SRS_PassengerBuckleSwitchStatus_S/1
  SRS_PassengerBuckleSwitchStatus_Convert/1 -> SRS_PassengerBuckleSwitchStatus_L/1
  SRS_PassengerBuckleSwitchStatus_Sub/1(Out1) -> SRS_PassengerBuckleSwitchStatus_Convert/1
  Demux/4 -> SRS_DriverBuckleSwitchStatus_Sub/1(In1), SRS_PassengerBuckleSwitchStatus_Sub/1(In1)
  SRS_PassengerBuckleSwitchStatus_sat/1 -> SRS_PassengerBuckleSwitchStatus_Out/1
  SRS_PassengerBuckleSwitchStatus_Ad/1 -> SRS_PassengerBuckleSwitchStatus_sat/1
  SRS_PassengerBuckleSwitchStatus_O/1 -> SRS_PassengerBuckleSwitchStatus_Ad/2
  SRS_PassengerBuckleSwitchStatus_F/1 -> SRS_PassengerBuckleSwitchStatus_Ad/1
